simulink model "pulse_detector_v4_fil_tb"  (R2022b)
settings: Solver=FixedStepDiscrete  StartTime=0.0  StopTime=SimTime  RelTol=1e-3
undefined symbols (not defined in the file): RxSignal
libraries: dspsrcs4 x2, hdlsllib x1
settings Model: DataTypeOverride=Off  Creator=cchung  LastModifiedBy=bsingh
settings SolverCC: AlgebraicLoopSolver=TrustRegion
settings DataIOCC: SaveOutput=off  SaveTime=off
settings OptimizationCC: BlockReduction=off  ConditionallyExecuteInputs=off  DefaultParameterBehavior=Inlined  InheritOutputTypeSmallerThanSingle=on  ReuseModelBlockBuffer=on
settings DebuggingCC: AlgebraicLoopMsg=error  SingleTaskRateTransMsg=error  UnconnectedInputMsg=warning  UnconnectedOutputMsg=warning  UnconnectedLineMsg=warning  PregeneratedLibrarySubsystemCodeDiagnostic=none  ArithmeticOperatorsInVariantConditions=warning
settings HardwareCC: ProdBitPerPointer=32  ProdBitPerSizeT=32  ProdBitPerPtrDiffT=32  ProdLargestAtomicFloat=None  ProdIntDivRoundTo=Undefined  ProdEndianess=Unspecified  ProdWordSize=32  ProdHWDeviceType=ASIC/FPGA->ASIC/FPGA  TargetBitPerPointer=64  TargetBitPerSizeT=64  TargetBitPerPtrDiffT=64  TargetLongLongMode=on  TargetIntDivRoundTo=Zero  TargetEndianess=LittleEndian  TargetWordSize=64  TargetHWDeviceType=Custom Processor->MATLAB Host Computer  ProdEqTarget=off
settings ModelReferenceCC: EnableRefExpFcnMdlSchedulingChecks=on
settings SFSimCC: SimUseLocalCustomCode=off  CustomCodeUndefinedFunction=UseInterfaceOnly
settings RTWCC: RTWUseLocalCustomCode=off  DLArmComputeVersion=19.05

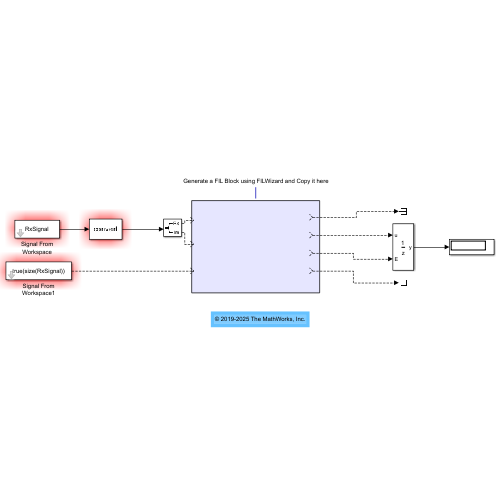
[thumbnail: Simulink's stored preview of the top-level diagram]
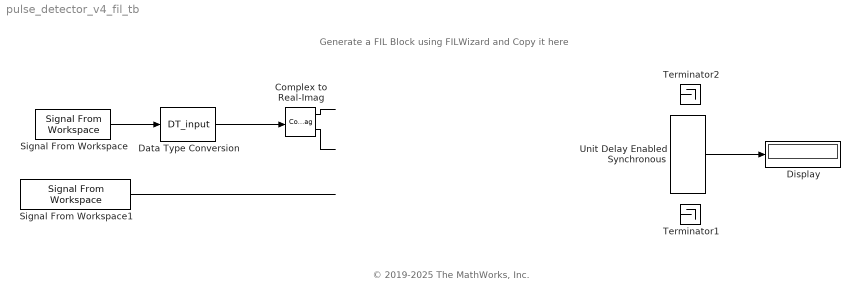
== system pulse_detector_v4_fil_tb ==
  note: Generate a FIL Block using FILWizard and Copy it here
  note: © 2019-2025 The MathWorks, Inc.
  Complex to Real-Imag : ComplexToRealImag
  Data Type Conversion : DataTypeConversion  OutDataTypeStr=DT_input  RndMeth=Nearest
  Display : Display
  Signal From Workspace : dspsrcs4/Signal From Workspace  X=RxSignal  Ts=1  nsamps=1  OutputAfterFinalValue=Setting to zero  ignoreOrWarnInputAndFrameLengths=off  OutputFrames=off
  Signal From Workspace1 : dspsrcs4/Signal From Workspace  X=true(size(RxSignal))  Ts=1  nsamps=1  OutputAfterFinalValue=Setting to zero  ignoreOrWarnInputAndFrameLengths=off  OutputFrames=off
  Terminator1 : Terminator
  Terminator2 : Terminator
  Unit Delay Enabled Synchronous : hdlsllib/Discrete/Unit Delay Enabled Synchronous  InitialCondition=0.0  SampleTime=-1
  wires:
  Unit Delay Enabled Synchronous/1 -> Display/1
  Signal From Workspace/1 -> Data Type Conversion/1
  ? -> Unit Delay Enabled Synchronous/1
  ? -> Unit Delay Enabled Synchronous/2
  Signal From Workspace1/1 -> ?
  ? -> Terminator1/1
  Data Type Conversion/1 -> Complex to Real-Imag/1
  ? -> Terminator2/1
  Complex to Real-Imag/1 -> ?
  Complex to Real-Imag/2 -> ?
